simulink model "VCU_CS75_12_30_test"  (R2014a)
settings: Solver=FixedStepDiscrete  StartTime=0.0  StopTime=25  FixedStep=0.0005  RelTol=1e-3
InitFcn:
  | PID_canshu
values from neighbouring files (symbols this model uses):
  D1 = ecucoder_cal(D1)    [PID_canshu.m]
  D2 = ecucoder_cal(D2)    [PID_canshu.m]
  D3 = ecucoder_cal(D3)    [PID_canshu.m]
  ErrorLimit = ecucoder_cal(ErrorLimit)    [PID_canshu.m]
  ErrorSumMax1 = ecucoder_cal(ErrorSumMax1)    [PID_canshu.m]
  ErrorSumMax2 = ecucoder_cal(ErrorSumMax2)    [PID_canshu.m]
  ErrorSumMax3 = ecucoder_cal(ErrorSumMax3)    [PID_canshu.m]
  I1 = ecucoder_cal(I1)    [PID_canshu.m]
  I2 = ecucoder_cal(I2)    [PID_canshu.m]
  I3 = ecucoder_cal(I3)    [PID_canshu.m]
  Limit1 = ecucoder_cal(Limit1)    [PID_canshu.m]
  Limit2 = ecucoder_cal(Limit2)    [PID_canshu.m]
  P1 = ecucoder_cal(P1)    [PID_canshu.m]
  P2 = ecucoder_cal(P2)    [PID_canshu.m]
  P3 = ecucoder_cal(P3)    [PID_canshu.m]
  T_buchang = ecucoder_cal(T_buchang)    [PID_canshu.m]
undefined symbols (not defined in the file or in its folder): ecucoder_acal, I_SW01_L, LaterlAngleCommand, LDW, RemoteAcclPosition
libraries: simulink x940, ec5744lib x41
(part 20 of 31)

== system VCU_CS75_12_30_test/长安CS75底盘程序，20ms一次/Output/Subsystem/TransmitMessages10/LAS_29D/LAS_HostLaneLeftStatus ==
  LAS_HostLaneLeftStatus : Inport
  Constant{1..2,4..8} (7 alike) : Constant  Value=0  OutDataTypeStr=uint8
  LAS_HostLaneLeftStatusRon : Rounding  Operator=round
  LAS_HostLaneLeftStatus_1sat : Saturate  UpperLimit=7  LowerLimit=0
  LAS_HostLaneLeftStatus_Convert : DataTypeConversion  OutDataTypeStr=uint8
  LAS_HostLaneLeftStatus_Convert1 : DataTypeConversion  OutDataTypeStr=uint32
  LAS_HostLaneLeftStatus_D : Product  Inputs=*/
  LAS_HostLaneLeftStatus_F : Constant  OutDataTypeStr=single
  LAS_HostLaneLeftStatus_L : simulink/Logic and Bit Operations/Bitwise Operator  logicop=AND  UseBitMask=on  BitMask=7  BitMaskRealWorld=Stored Integer
  LAS_HostLaneLeftStatus_O : Constant  Value=0  OutDataTypeStr=single
  LAS_HostLaneLeftStatus_S : ArithShift
  LAS_HostLaneLeftStatus_sat : Saturate  UpperLimit=0  LowerLimit=0
  LAS_HostLaneLeftStatus_st : Sum  Inputs=+-
  output1 : Outport
  output2 : Outport  Port=2
  output3 : Outport  Port=3
  output4 : Outport  Port=4
  output5 : Outport  Port=5
  output6 : Outport  Port=6
  output7 : Outport  Port=7
  output8 : Outport  Port=8
  wires:
  LAS_HostLaneLeftStatus/1 -> LAS_HostLaneLeftStatus_sat/1
  LAS_HostLaneLeftStatus_sat/1 -> LAS_HostLaneLeftStatus_st/1
  LAS_HostLaneLeftStatus_O/1 -> LAS_HostLaneLeftStatus_st/2
  LAS_HostLaneLeftStatus_st/1 -> LAS_HostLaneLeftStatus_D/1
  LAS_HostLaneLeftStatus_F/1 -> LAS_HostLaneLeftStatus_D/2
  LAS_HostLaneLeftStatus_D/1 -> LAS_HostLaneLeftStatusRon/1
  LAS_HostLaneLeftStatusRon/1 -> LAS_HostLaneLeftStatus_S/1
  LAS_HostLaneLeftStatus_S/1 -> LAS_HostLaneLeftStatus_1sat/1
  LAS_HostLaneLeftStatus_1sat/1 -> LAS_HostLaneLeftStatus_Convert1/1
  LAS_HostLaneLeftStatus_Convert1/1 -> LAS_HostLaneLeftStatus_L/1
  LAS_HostLaneLeftStatus_L/1 -> LAS_HostLaneLeftStatus_Convert/1
  LAS_HostLaneLeftStatus_Convert/1 -> output3/1
  Constant1/1 -> output1/1
  Constant2/1 -> output2/1
  Constant4/1 -> output4/1
  Constant5/1 -> output5/1
  Constant6/1 -> output6/1
  Constant7/1 -> output7/1
  Constant8/1 -> output8/1

== system VCU_CS75_12_30_test/长安CS75底盘程序，20ms一次/Output/Subsystem/TransmitMessages10/LAS_29D/LAS_HostLaneRightStatus ==
  LAS_HostLaneRightStatus : Inport
  Constant{1..3,5..8} (7 alike) : Constant  Value=0  OutDataTypeStr=uint8
  LAS_HostLaneRightStatusRon : Rounding  Operator=round
  LAS_HostLaneRightStatus_1sat : Saturate  UpperLimit=7  LowerLimit=0
  LAS_HostLaneRightStatus_Convert : DataTypeConversion  OutDataTypeStr=uint8
  LAS_HostLaneRightStatus_Convert1 : DataTypeConversion  OutDataTypeStr=uint32
  LAS_HostLaneRightStatus_D : Product  Inputs=*/
  LAS_HostLaneRightStatus_F : Constant  OutDataTypeStr=single
  LAS_HostLaneRightStatus_L : simulink/Logic and Bit Operations/Bitwise Operator  logicop=AND  UseBitMask=on  BitMask=7  BitMaskRealWorld=Stored Integer
  LAS_HostLaneRightStatus_O : Constant  Value=0  OutDataTypeStr=single
  LAS_HostLaneRightStatus_S : ArithShift
  LAS_HostLaneRightStatus_sat : Saturate  UpperLimit=0  LowerLimit=0
  LAS_HostLaneRightStatus_st : Sum  Inputs=+-
  output1 : Outport
  output2 : Outport  Port=2
  output3 : Outport  Port=3
  output4 : Outport  Port=4
  output5 : Outport  Port=5
  output6 : Outport  Port=6
  output7 : Outport  Port=7
  output8 : Outport  Port=8
  wires:
  LAS_HostLaneRightStatus/1 -> LAS_HostLaneRightStatus_sat/1
  LAS_HostLaneRightStatus_sat/1 -> LAS_HostLaneRightStatus_st/1
  LAS_HostLaneRightStatus_O/1 -> LAS_HostLaneRightStatus_st/2
  LAS_HostLaneRightStatus_st/1 -> LAS_HostLaneRightStatus_D/1
  LAS_HostLaneRightStatus_F/1 -> LAS_HostLaneRightStatus_D/2
  LAS_HostLaneRightStatus_D/1 -> LAS_HostLaneRightStatusRon/1
  LAS_HostLaneRightStatusRon/1 -> LAS_HostLaneRightStatus_S/1
  LAS_HostLaneRightStatus_S/1 -> LAS_HostLaneRightStatus_1sat/1
  LAS_HostLaneRightStatus_1sat/1 -> LAS_HostLaneRightStatus_Convert1/1
  LAS_HostLaneRightStatus_Convert1/1 -> LAS_HostLaneRightStatus_L/1
  LAS_HostLaneRightStatus_L/1 -> LAS_HostLaneRightStatus_Convert/1
  LAS_HostLaneRightStatus_Convert/1 -> output4/1
  Constant1/1 -> output1/1
  Constant2/1 -> output2/1
  Constant3/1 -> output3/1
  Constant5/1 -> output5/1
  Constant6/1 -> output6/1
  Constant7/1 -> output7/1
  Constant8/1 -> output8/1

== system VCU_CS75_12_30_test/长安CS75底盘程序，20ms一次/Output/Subsystem/TransmitMessages10/LAS_29D/LAS_IACCEnableStatus ==
  LAS_IACCEnableStatus : Inport
  Constant{1..6,8} (7 alike) : Constant  Value=0  OutDataTypeStr=uint8
  LAS_IACCEnableStatusRon : Rounding  Operator=round
  LAS_IACCEnableStatus_1sat : Saturate  UpperLimit=48  LowerLimit=0
  LAS_IACCEnableStatus_Convert : DataTypeConversion  OutDataTypeStr=uint8
  LAS_IACCEnableStatus_Convert1 : DataTypeConversion  OutDataTypeStr=uint32
  LAS_IACCEnableStatus_D : Product  Inputs=*/
  LAS_IACCEnableStatus_F : Constant  OutDataTypeStr=single
  LAS_IACCEnableStatus_L : simulink/Logic and Bit Operations/Bitwise Operator  logicop=AND  UseBitMask=on  BitMask=48  BitMaskRealWorld=Stored Integer
  LAS_IACCEnableStatus_O : Constant  Value=0  OutDataTypeStr=single
  LAS_IACCEnableStatus_S : ArithShift  BitShiftNumber=-4
  LAS_IACCEnableStatus_sat : Saturate  UpperLimit=3  LowerLimit=0
  LAS_IACCEnableStatus_st : Sum  Inputs=+-
  output1 : Outport
  output2 : Outport  Port=2
  output3 : Outport  Port=3
  output4 : Outport  Port=4
  output5 : Outport  Port=5
  output6 : Outport  Port=6
  output7 : Outport  Port=7
  output8 : Outport  Port=8
  wires:
  LAS_IACCEnableStatus/1 -> LAS_IACCEnableStatus_sat/1
  LAS_IACCEnableStatus_sat/1 -> LAS_IACCEnableStatus_st/1
  LAS_IACCEnableStatus_O/1 -> LAS_IACCEnableStatus_st/2
  LAS_IACCEnableStatus_st/1 -> LAS_IACCEnableStatus_D/1
  LAS_IACCEnableStatus_F/1 -> LAS_IACCEnableStatus_D/2
  LAS_IACCEnableStatus_D/1 -> LAS_IACCEnableStatusRon/1
  LAS_IACCEnableStatusRon/1 -> LAS_IACCEnableStatus_S/1
  LAS_IACCEnableStatus_S/1 -> LAS_IACCEnableStatus_1sat/1
  LAS_IACCEnableStatus_1sat/1 -> LAS_IACCEnableStatus_Convert1/1
  LAS_IACCEnableStatus_Convert1/1 -> LAS_IACCEnableStatus_L/1
  LAS_IACCEnableStatus_L/1 -> LAS_IACCEnableStatus_Convert/1
  LAS_IACCEnableStatus_Convert/1 -> output7/1
  Constant1/1 -> output1/1
  Constant2/1 -> output2/1
  Constant3/1 -> output3/1
  Constant4/1 -> output4/1
  Constant5/1 -> output5/1
  Constant6/1 -> output6/1
  Constant8/1 -> output8/1

== system VCU_CS75_12_30_test/长安CS75底盘程序，20ms一次/Output/Subsystem/TransmitMessages10/LAS_29D/LAS_LASModeSelectionStatus ==
  LAS_LASModeSelectionStatus : Inport
  Constant{2..8} (7 alike) : Constant  Value=0  OutDataTypeStr=uint8
  LAS_LASModeSelectionStatusRon : Rounding  Operator=round
  LAS_LASModeSelectionStatus_1sat : Saturate  UpperLimit=56  LowerLimit=0
  LAS_LASModeSelectionStatus_Convert : DataTypeConversion  OutDataTypeStr=uint8
  LAS_LASModeSelectionStatus_Convert1 : DataTypeConversion  OutDataTypeStr=uint32
  LAS_LASModeSelectionStatus_D : Product  Inputs=*/
  LAS_LASModeSelectionStatus_F : Constant  OutDataTypeStr=single
  LAS_LASModeSelectionStatus_L : simulink/Logic and Bit Operations/Bitwise Operator  logicop=AND  UseBitMask=on  BitMask=56  BitMaskRealWorld=Stored Integer
  LAS_LASModeSelectionStatus_O : Constant  Value=0  OutDataTypeStr=single
  LAS_LASModeSelectionStatus_S : ArithShift  BitShiftNumber=-3
  LAS_LASModeSelectionStatus_sat : Saturate  UpperLimit=7  LowerLimit=0
  LAS_LASModeSelectionStatus_st : Sum  Inputs=+-
  output1 : Outport
  output2 : Outport  Port=2
  output3 : Outport  Port=3
  output4 : Outport  Port=4
  output5 : Outport  Port=5
  output6 : Outport  Port=6
  output7 : Outport  Port=7
  output8 : Outport  Port=8
  wires:
  LAS_LASModeSelectionStatus/1 -> LAS_LASModeSelectionStatus_sat/1
  LAS_LASModeSelectionStatus_sat/1 -> LAS_LASModeSelectionStatus_st/1
  LAS_LASModeSelectionStatus_O/1 -> LAS_LASModeSelectionStatus_st/2
  LAS_LASModeSelectionStatus_st/1 -> LAS_LASModeSelectionStatus_D/1
  LAS_LASModeSelectionStatus_F/1 -> LAS_LASModeSelectionStatus_D/2
  LAS_LASModeSelectionStatus_D/1 -> LAS_LASModeSelectionStatusRon/1
  LAS_LASModeSelectionStatusRon/1 -> LAS_LASModeSelectionStatus_S/1
  LAS_LASModeSelectionStatus_S/1 -> LAS_LASModeSelectionStatus_1sat/1
  LAS_LASModeSelectionStatus_1sat/1 -> LAS_LASModeSelectionStatus_Convert1/1
  LAS_LASModeSelectionStatus_Convert1/1 -> LAS_LASModeSelectionStatus_L/1
  LAS_LASModeSelectionStatus_L/1 -> LAS_LASModeSelectionStatus_Convert/1
  LAS_LASModeSelectionStatus_Convert/1 -> output1/1
  Constant2/1 -> output2/1
  Constant3/1 -> output3/1
  Constant4/1 -> output4/1
  Constant5/1 -> output5/1
  Constant6/1 -> output6/1
  Constant7/1 -> output7/1
  Constant8/1 -> output8/1

== system VCU_CS75_12_30_test/长安CS75底盘程序，20ms一次/Output/Subsystem/TransmitMessages10/LAS_29D/LAS_LASWarningModeSelectionSts ==
  LAS_LASWarningModeSelectionSts : Inport
  Constant{3..8} (6 alike) : Constant  Value=0  OutDataTypeStr=uint8
  LAS_LASWarningModeSelectionStsBitCov : DataTypeConversion  OutDataTypeStr=uint8
  LAS_LASWarningModeSelectionStsCOV : DataTypeConversion  OutDataTypeStr=uint8
  LAS_LASWarningModeSelectionStsRon : Rounding  Operator=round
  LAS_LASWarningModeSelectionSts_1sat : Saturate  UpperLimit=448  LowerLimit=0
  LAS_LASWarningModeSelectionSts_And : simulink/Logic and Bit Operations/Bitwise Operator  logicop=AND  UseBitMask=off  NumInputPorts=2  BitMask=bin2dec('11011001')  BitMaskRealWorld=Stored Integer
  LAS_LASWarningModeSelectionSts_And_C : Constant  Value=255  OutDataTypeStr=uint32
  LAS_LASWarningModeSelectionSts_Convert : DataTypeConversion  OutDataTypeStr=uint32
  LAS_LASWarningModeSelectionSts_D : Product  Inputs=*/
  LAS_LASWarningModeSelectionSts_D1 : Product  Inputs=*/
  LAS_LASWarningModeSelectionSts_F : Constant  OutDataTypeStr=single
  LAS_LASWarningModeSelectionSts_L : simulink/Logic and Bit Operations/Bitwise Operator  logicop=AND  UseBitMask=on  BitMask=448  BitMaskRealWorld=Stored Integer
  LAS_LASWarningModeSelectionSts_O : Constant  Value=0  OutDataTypeStr=single
  LAS_LASWarningModeSelectionSts_S : ArithShift  BitShiftNumber=-6
  LAS_LASWarningModeSelectionSts_sat : Saturate  UpperLimit=7  LowerLimit=0
  LAS_LASWarningModeSelectionSts_st : Sum  Inputs=+-
  LAS_LASWarningModeSelectionStsoutput1_C : Constant  Value=256
  output1 : Outport
  output2 : Outport  Port=2
  output3 : Outport  Port=3
  output4 : Outport  Port=4
  output5 : Outport  Port=5
  output6 : Outport  Port=6
  output7 : Outport  Port=7
  output8 : Outport  Port=8
  wires:
  LAS_LASWarningModeSelectionSts/1 -> LAS_LASWarningModeSelectionSts_sat/1
  LAS_LASWarningModeSelectionSts_sat/1 -> LAS_LASWarningModeSelectionSts_st/1
  LAS_LASWarningModeSelectionSts_O/1 -> LAS_LASWarningModeSelectionSts_st/2
  LAS_LASWarningModeSelectionSts_st/1 -> LAS_LASWarningModeSelectionSts_D/1
  LAS_LASWarningModeSelectionSts_F/1 -> LAS_LASWarningModeSelectionSts_D/2
  LAS_LASWarningModeSelectionSts_D/1 -> LAS_LASWarningModeSelectionStsRon/1
  LAS_LASWarningModeSelectionStsRon/1 -> LAS_LASWarningModeSelectionSts_S/1
  LAS_LASWarningModeSelectionSts_S/1 -> LAS_LASWarningModeSelectionSts_1sat/1
  LAS_LASWarningModeSelectionSts_1sat/1 -> LAS_LASWarningModeSelectionSts_Convert/1
  LAS_LASWarningModeSelectionSts_Convert/1 -> LAS_LASWarningModeSelectionSts_L/1
  LAS_LASWarningModeSelectionSts_L/1 -> LAS_LASWarningModeSelectionSts_D1/1, LAS_LASWarningModeSelectionSts_And/1
  LAS_LASWarningModeSelectionStsoutput1_C/1 -> LAS_LASWarningModeSelectionSts_D1/2
  LAS_LASWarningModeSelectionSts_D1/1 -> LAS_LASWarningModeSelectionStsCOV/1
  LAS_LASWarningModeSelectionStsCOV/1 -> output1/1
  LAS_LASWarningModeSelectionSts_And_C/1 -> LAS_LASWarningModeSelectionSts_And/2
  LAS_LASWarningModeSelectionSts_And/1 -> LAS_LASWarningModeSelectionStsBitCov/1
  LAS_LASWarningModeSelectionStsBitCov/1 -> output2/1
  Constant3/1 -> output3/1
  Constant4/1 -> output4/1
  Constant5/1 -> output5/1
  Constant6/1 -> output6/1
  Constant7/1 -> output7/1
  Constant8/1 -> output8/1

== system VCU_CS75_12_30_test/长安CS75底盘程序，20ms一次/Output/Subsystem/TransmitMessages10/LAS_29D/LAS_LDWShakeLevStatus ==
  LAS_LDWShakeLevStatus : Inport
  Constant{1,3..8} (7 alike) : Constant  Value=0  OutDataTypeStr=uint8
  LAS_LDWShakeLevStatusRon : Rounding  Operator=round
  LAS_LDWShakeLevStatus_1sat : Saturate  UpperLimit=48  LowerLimit=0
  LAS_LDWShakeLevStatus_Convert : DataTypeConversion  OutDataTypeStr=uint8
  LAS_LDWShakeLevStatus_Convert1 : DataTypeConversion  OutDataTypeStr=uint32
  LAS_LDWShakeLevStatus_D : Product  Inputs=*/
  LAS_LDWShakeLevStatus_F : Constant  OutDataTypeStr=single
  LAS_LDWShakeLevStatus_L : simulink/Logic and Bit Operations/Bitwise Operator  logicop=AND  UseBitMask=on  BitMask=48  BitMaskRealWorld=Stored Integer
  LAS_LDWShakeLevStatus_O : Constant  Value=0  OutDataTypeStr=single
  LAS_LDWShakeLevStatus_S : ArithShift  BitShiftNumber=-4
  LAS_LDWShakeLevStatus_sat : Saturate  UpperLimit=3  LowerLimit=0
  LAS_LDWShakeLevStatus_st : Sum  Inputs=+-
  output1 : Outport
  output2 : Outport  Port=2
  output3 : Outport  Port=3
  output4 : Outport  Port=4
  output5 : Outport  Port=5
  output6 : Outport  Port=6
  output7 : Outport  Port=7
  output8 : Outport  Port=8
  wires:
  LAS_LDWShakeLevStatus/1 -> LAS_LDWShakeLevStatus_sat/1
  LAS_LDWShakeLevStatus_sat/1 -> LAS_LDWShakeLevStatus_st/1
  LAS_LDWShakeLevStatus_O/1 -> LAS_LDWShakeLevStatus_st/2
  LAS_LDWShakeLevStatus_st/1 -> LAS_LDWShakeLevStatus_D/1
  LAS_LDWShakeLevStatus_F/1 -> LAS_LDWShakeLevStatus_D/2
  LAS_LDWShakeLevStatus_D/1 -> LAS_LDWShakeLevStatusRon/1
  LAS_LDWShakeLevStatusRon/1 -> LAS_LDWShakeLevStatus_S/1
  LAS_LDWShakeLevStatus_S/1 -> LAS_LDWShakeLevStatus_1sat/1
  LAS_LDWShakeLevStatus_1sat/1 -> LAS_LDWShakeLevStatus_Convert1/1
  LAS_LDWShakeLevStatus_Convert1/1 -> LAS_LDWShakeLevStatus_L/1
  LAS_LDWShakeLevStatus_L/1 -> LAS_LDWShakeLevStatus_Convert/1
  LAS_LDWShakeLevStatus_Convert/1 -> output2/1
  Constant1/1 -> output1/1
  Constant3/1 -> output3/1
  Constant4/1 -> output4/1
  Constant5/1 -> output5/1
  Constant6/1 -> output6/1
  Constant7/1 -> output7/1
  Constant8/1 -> output8/1

== system VCU_CS75_12_30_test/长安CS75底盘程序，20ms一次/Output/Subsystem/TransmitMessages10/LAS_29D/LAS_LLaneMarkerType ==
  LAS_LLaneMarkerType : Inport
  Constant{1..4,6..8} (7 alike) : Constant  Value=0  OutDataTypeStr=uint8
  LAS_LLaneMarkerTypeRon : Rounding  Operator=round
  LAS_LLaneMarkerType_1sat : Saturate  UpperLimit=7  LowerLimit=0
  LAS_LLaneMarkerType_Convert : DataTypeConversion  OutDataTypeStr=uint8
  LAS_LLaneMarkerType_Convert1 : DataTypeConversion  OutDataTypeStr=uint32
  LAS_LLaneMarkerType_D : Product  Inputs=*/
  LAS_LLaneMarkerType_F : Constant  OutDataTypeStr=single
  LAS_LLaneMarkerType_L : simulink/Logic and Bit Operations/Bitwise Operator  logicop=AND  UseBitMask=on  BitMask=7  BitMaskRealWorld=Stored Integer
  LAS_LLaneMarkerType_O : Constant  Value=0  OutDataTypeStr=single
  LAS_LLaneMarkerType_S : ArithShift
  LAS_LLaneMarkerType_sat : Saturate  UpperLimit=7  LowerLimit=0
  LAS_LLaneMarkerType_st : Sum  Inputs=+-
  output1 : Outport
  output2 : Outport  Port=2
  output3 : Outport  Port=3
  output4 : Outport  Port=4
  output5 : Outport  Port=5
  output6 : Outport  Port=6
  output7 : Outport  Port=7
  output8 : Outport  Port=8
  wires:
  LAS_LLaneMarkerType/1 -> LAS_LLaneMarkerType_sat/1
  LAS_LLaneMarkerType_sat/1 -> LAS_LLaneMarkerType_st/1
  LAS_LLaneMarkerType_O/1 -> LAS_LLaneMarkerType_st/2
  LAS_LLaneMarkerType_st/1 -> LAS_LLaneMarkerType_D/1
  LAS_LLaneMarkerType_F/1 -> LAS_LLaneMarkerType_D/2
  LAS_LLaneMarkerType_D/1 -> LAS_LLaneMarkerTypeRon/1
  LAS_LLaneMarkerTypeRon/1 -> LAS_LLaneMarkerType_S/1
  LAS_LLaneMarkerType_S/1 -> LAS_LLaneMarkerType_1sat/1
  LAS_LLaneMarkerType_1sat/1 -> LAS_LLaneMarkerType_Convert1/1
  LAS_LLaneMarkerType_Convert1/1 -> LAS_LLaneMarkerType_L/1
  LAS_LLaneMarkerType_L/1 -> LAS_LLaneMarkerType_Convert/1
  LAS_LLaneMarkerType_Convert/1 -> output5/1
  Constant1/1 -> output1/1
  Constant2/1 -> output2/1
  Constant3/1 -> output3/1
  Constant4/1 -> output4/1
  Constant6/1 -> output6/1
  Constant7/1 -> output7/1
  Constant8/1 -> output8/1

== system VCU_CS75_12_30_test/长安CS75底盘程序，20ms一次/Output/Subsystem/TransmitMessages10/LAS_29D/LAS_LdwSensitivityStatus ==
  LAS_LdwSensitivityStatus : Inport
  Constant{2..8} (7 alike) : Constant  Value=0  OutDataTypeStr=uint8
  LAS_LdwSensitivityStatusRon : Rounding  Operator=round
  LAS_LdwSensitivityStatus_1sat : Saturate  UpperLimit=192  LowerLimit=0
  LAS_LdwSensitivityStatus_Convert : DataTypeConversion  OutDataTypeStr=uint8
  LAS_LdwSensitivityStatus_Convert1 : DataTypeConversion  OutDataTypeStr=uint32
  LAS_LdwSensitivityStatus_D : Product  Inputs=*/
  LAS_LdwSensitivityStatus_F : Constant  OutDataTypeStr=single
  LAS_LdwSensitivityStatus_L : simulink/Logic and Bit Operations/Bitwise Operator  logicop=AND  UseBitMask=on  BitMask=192  BitMaskRealWorld=Stored Integer
  LAS_LdwSensitivityStatus_O : Constant  Value=0  OutDataTypeStr=single
  LAS_LdwSensitivityStatus_S : ArithShift  BitShiftNumber=-6
  LAS_LdwSensitivityStatus_sat : Saturate  UpperLimit=3  LowerLimit=0
  LAS_LdwSensitivityStatus_st : Sum  Inputs=+-
  output1 : Outport
  output2 : Outport  Port=2
  output3 : Outport  Port=3
  output4 : Outport  Port=4
  output5 : Outport  Port=5
  output6 : Outport  Port=6
  output7 : Outport  Port=7
  output8 : Outport  Port=8
  wires:
  LAS_LdwSensitivityStatus/1 -> LAS_LdwSensitivityStatus_sat/1
  LAS_LdwSensitivityStatus_sat/1 -> LAS_LdwSensitivityStatus_st/1
  LAS_LdwSensitivityStatus_O/1 -> LAS_LdwSensitivityStatus_st/2
  LAS_LdwSensitivityStatus_st/1 -> LAS_LdwSensitivityStatus_D/1
  LAS_LdwSensitivityStatus_F/1 -> LAS_LdwSensitivityStatus_D/2
  LAS_LdwSensitivityStatus_D/1 -> LAS_LdwSensitivityStatusRon/1
  LAS_LdwSensitivityStatusRon/1 -> LAS_LdwSensitivityStatus_S/1
  LAS_LdwSensitivityStatus_S/1 -> LAS_LdwSensitivityStatus_1sat/1
  LAS_LdwSensitivityStatus_1sat/1 -> LAS_LdwSensitivityStatus_Convert1/1
  LAS_LdwSensitivityStatus_Convert1/1 -> LAS_LdwSensitivityStatus_L/1
  LAS_LdwSensitivityStatus_L/1 -> LAS_LdwSensitivityStatus_Convert/1
  LAS_LdwSensitivityStatus_Convert/1 -> output1/1
  Constant2/1 -> output2/1
  Constant3/1 -> output3/1
  Constant4/1 -> output4/1
  Constant5/1 -> output5/1
  Constant6/1 -> output6/1
  Constant7/1 -> output7/1
  Constant8/1 -> output8/1

== system VCU_CS75_12_30_test/长安CS75底盘程序，20ms一次/Output/Subsystem/TransmitMessages10/LAS_29D/LAS_OverspeedSoundWarning ==
  LAS_OverspeedSoundWarning : Inport
  Constant{1..3,5..8} (7 alike) : Constant  Value=0  OutDataTypeStr=uint8
  LAS_OverspeedSoundWarningRon : Rounding  Operator=round
  LAS_OverspeedSoundWarning_1sat : Saturate  UpperLimit=192  LowerLimit=0
  LAS_OverspeedSoundWarning_Convert : DataTypeConversion  OutDataTypeStr=uint8
  LAS_OverspeedSoundWarning_Convert1 : DataTypeConversion  OutDataTypeStr=uint32
  LAS_OverspeedSoundWarning_D : Product  Inputs=*/
  LAS_OverspeedSoundWarning_F : Constant  OutDataTypeStr=single
  LAS_OverspeedSoundWarning_L : simulink/Logic and Bit Operations/Bitwise Operator  logicop=AND  UseBitMask=on  BitMask=192  BitMaskRealWorld=Stored Integer
  LAS_OverspeedSoundWarning_O : Constant  Value=0  OutDataTypeStr=single
  LAS_OverspeedSoundWarning_S : ArithShift  BitShiftNumber=-6
  LAS_OverspeedSoundWarning_sat : Saturate  UpperLimit=3  LowerLimit=0
  LAS_OverspeedSoundWarning_st : Sum  Inputs=+-
  output1 : Outport
  output2 : Outport  Port=2
  output3 : Outport  Port=3
  output4 : Outport  Port=4
  output5 : Outport  Port=5
  output6 : Outport  Port=6
  output7 : Outport  Port=7
  output8 : Outport  Port=8
  wires:
  LAS_OverspeedSoundWarning/1 -> LAS_OverspeedSoundWarning_sat/1
  LAS_OverspeedSoundWarning_sat/1 -> LAS_OverspeedSoundWarning_st/1
  LAS_OverspeedSoundWarning_O/1 -> LAS_OverspeedSoundWarning_st/2
  LAS_OverspeedSoundWarning_st/1 -> LAS_OverspeedSoundWarning_D/1
  LAS_OverspeedSoundWarning_F/1 -> LAS_OverspeedSoundWarning_D/2
  LAS_OverspeedSoundWarning_D/1 -> LAS_OverspeedSoundWarningRon/1
  LAS_OverspeedSoundWarningRon/1 -> LAS_OverspeedSoundWarning_S/1
  LAS_OverspeedSoundWarning_S/1 -> LAS_OverspeedSoundWarning_1sat/1
  LAS_OverspeedSoundWarning_1sat/1 -> LAS_OverspeedSoundWarning_Convert1/1
  LAS_OverspeedSoundWarning_Convert1/1 -> LAS_OverspeedSoundWarning_L/1
  LAS_OverspeedSoundWarning_L/1 -> LAS_OverspeedSoundWarning_Convert/1
  LAS_OverspeedSoundWarning_Convert/1 -> output4/1
  Constant1/1 -> output1/1
  Constant2/1 -> output2/1
  Constant3/1 -> output3/1
  Constant5/1 -> output5/1
  Constant6/1 -> output6/1
  Constant7/1 -> output7/1
  Constant8/1 -> output8/1

== system VCU_CS75_12_30_test/长安CS75底盘程序，20ms一次/Output/Subsystem/TransmitMessages10/LAS_29D/LAS_OverspeedSoundWarningEnSt ==
  LAS_OverspeedSoundWarningEnSt : Inport
  Constant{1,3..8} (7 alike) : Constant  Value=0  OutDataTypeStr=uint8
  LAS_OverspeedSoundWarningEnStRon : Rounding  Operator=round
  LAS_OverspeedSoundWarningEnSt_1sat : Saturate  UpperLimit=3  LowerLimit=0
  LAS_OverspeedSoundWarningEnSt_Convert : DataTypeConversion  OutDataTypeStr=uint8
  LAS_OverspeedSoundWarningEnSt_Convert1 : DataTypeConversion  OutDataTypeStr=uint32
  LAS_OverspeedSoundWarningEnSt_D : Product  Inputs=*/
  LAS_OverspeedSoundWarningEnSt_F : Constant  OutDataTypeStr=single
  LAS_OverspeedSoundWarningEnSt_L : simulink/Logic and Bit Operations/Bitwise Operator  logicop=AND  UseBitMask=on  BitMask=3  BitMaskRealWorld=Stored Integer
  LAS_OverspeedSoundWarningEnSt_O : Constant  Value=0  OutDataTypeStr=single
  LAS_OverspeedSoundWarningEnSt_S : ArithShift
  LAS_OverspeedSoundWarningEnSt_sat : Saturate  UpperLimit=3  LowerLimit=0
  LAS_OverspeedSoundWarningEnSt_st : Sum  Inputs=+-
  output1 : Outport
  output2 : Outport  Port=2
  output3 : Outport  Port=3
  output4 : Outport  Port=4
  output5 : Outport  Port=5
  output6 : Outport  Port=6
  output7 : Outport  Port=7
  output8 : Outport  Port=8
  wires:
  LAS_OverspeedSoundWarningEnSt/1 -> LAS_OverspeedSoundWarningEnSt_sat/1
  LAS_OverspeedSoundWarningEnSt_sat/1 -> LAS_OverspeedSoundWarningEnSt_st/1
  LAS_OverspeedSoundWarningEnSt_O/1 -> LAS_OverspeedSoundWarningEnSt_st/2
  LAS_OverspeedSoundWarningEnSt_st/1 -> LAS_OverspeedSoundWarningEnSt_D/1
  LAS_OverspeedSoundWarningEnSt_F/1 -> LAS_OverspeedSoundWarningEnSt_D/2
  LAS_OverspeedSoundWarningEnSt_D/1 -> LAS_OverspeedSoundWarningEnStRon/1
  LAS_OverspeedSoundWarningEnStRon/1 -> LAS_OverspeedSoundWarningEnSt_S/1
  LAS_OverspeedSoundWarningEnSt_S/1 -> LAS_OverspeedSoundWarningEnSt_1sat/1
  LAS_OverspeedSoundWarningEnSt_1sat/1 -> LAS_OverspeedSoundWarningEnSt_Convert1/1
  LAS_OverspeedSoundWarningEnSt_Convert1/1 -> LAS_OverspeedSoundWarningEnSt_L/1
  LAS_OverspeedSoundWarningEnSt_L/1 -> LAS_OverspeedSoundWarningEnSt_Convert/1
  LAS_OverspeedSoundWarningEnSt_Convert/1 -> output2/1
  Constant1/1 -> output1/1
  Constant3/1 -> output3/1
  Constant4/1 -> output4/1
  Constant5/1 -> output5/1
  Constant6/1 -> output6/1
  Constant7/1 -> output7/1
  Constant8/1 -> output8/1

== system VCU_CS75_12_30_test/长安CS75底盘程序，20ms一次/Output/Subsystem/TransmitMessages10/LAS_29D/LAS_OverspeedVisualWarning ==
  LAS_OverspeedVisualWarning : Inport
  Constant{1..4,6..8} (7 alike) : Constant  Value=0  OutDataTypeStr=uint8
  LAS_OverspeedVisualWarningRon : Rounding  Operator=round
  LAS_OverspeedVisualWarning_1sat : Saturate  UpperLimit=192  LowerLimit=0
  LAS_OverspeedVisualWarning_Convert : DataTypeConversion  OutDataTypeStr=uint8
  LAS_OverspeedVisualWarning_Convert1 : DataTypeConversion  OutDataTypeStr=uint32
  LAS_OverspeedVisualWarning_D : Product  Inputs=*/
  LAS_OverspeedVisualWarning_F : Constant  OutDataTypeStr=single
  LAS_OverspeedVisualWarning_L : simulink/Logic and Bit Operations/Bitwise Operator  logicop=AND  UseBitMask=on  BitMask=192  BitMaskRealWorld=Stored Integer
  LAS_OverspeedVisualWarning_O : Constant  Value=0  OutDataTypeStr=single
  LAS_OverspeedVisualWarning_S : ArithShift  BitShiftNumber=-6
  LAS_OverspeedVisualWarning_sat : Saturate  UpperLimit=3  LowerLimit=0
  LAS_OverspeedVisualWarning_st : Sum  Inputs=+-
  output1 : Outport
  output2 : Outport  Port=2
  output3 : Outport  Port=3
  output4 : Outport  Port=4
  output5 : Outport  Port=5
  output6 : Outport  Port=6
  output7 : Outport  Port=7
  output8 : Outport  Port=8
  wires:
  LAS_OverspeedVisualWarning/1 -> LAS_OverspeedVisualWarning_sat/1
  LAS_OverspeedVisualWarning_sat/1 -> LAS_OverspeedVisualWarning_st/1
  LAS_OverspeedVisualWarning_O/1 -> LAS_OverspeedVisualWarning_st/2
  LAS_OverspeedVisualWarning_st/1 -> LAS_OverspeedVisualWarning_D/1
  LAS_OverspeedVisualWarning_F/1 -> LAS_OverspeedVisualWarning_D/2
  LAS_OverspeedVisualWarning_D/1 -> LAS_OverspeedVisualWarningRon/1
  LAS_OverspeedVisualWarningRon/1 -> LAS_OverspeedVisualWarning_S/1
  LAS_OverspeedVisualWarning_S/1 -> LAS_OverspeedVisualWarning_1sat/1
  LAS_OverspeedVisualWarning_1sat/1 -> LAS_OverspeedVisualWarning_Convert1/1
  LAS_OverspeedVisualWarning_Convert1/1 -> LAS_OverspeedVisualWarning_L/1
  LAS_OverspeedVisualWarning_L/1 -> LAS_OverspeedVisualWarning_Convert/1
  LAS_OverspeedVisualWarning_Convert/1 -> output5/1
  Constant1/1 -> output1/1
  Constant2/1 -> output2/1
  Constant3/1 -> output3/1
  Constant4/1 -> output4/1
  Constant6/1 -> output6/1
  Constant7/1 -> output7/1
  Constant8/1 -> output8/1

== system VCU_CS75_12_30_test/长安CS75底盘程序，20ms一次/Output/Subsystem/TransmitMessages10/LAS_29D/LAS_OverspeedWarningEnableStatus ==
  LAS_OverspeedWarningEnableStatus : Inport
  Constant{1..3,5..8} (7 alike) : Constant  Value=0  OutDataTypeStr=uint8
  LAS_OverspeedWarningEnableStatusRon : Rounding  Operator=round
  LAS_OverspeedWarningEnableStatus_1sat : Saturate  UpperLimit=48  LowerLimit=0
  LAS_OverspeedWarningEnableStatus_Convert : DataTypeConversion  OutDataTypeStr=uint8
  LAS_OverspeedWarningEnableStatus_Convert1 : DataTypeConversion  OutDataTypeStr=uint32
  LAS_OverspeedWarningEnableStatus_D : Product  Inputs=*/
  LAS_OverspeedWarningEnableStatus_F : Constant  OutDataTypeStr=single
  LAS_OverspeedWarningEnableStatus_L : simulink/Logic and Bit Operations/Bitwise Operator  logicop=AND  UseBitMask=on  BitMask=48  BitMaskRealWorld=Stored Integer
  LAS_OverspeedWarningEnableStatus_O : Constant  Value=0  OutDataTypeStr=single
  LAS_OverspeedWarningEnableStatus_S : ArithShift  BitShiftNumber=-4
  LAS_OverspeedWarningEnableStatus_sat : Saturate  UpperLimit=3  LowerLimit=0
  LAS_OverspeedWarningEnableStatus_st : Sum  Inputs=+-
  output1 : Outport
  output2 : Outport  Port=2
  output3 : Outport  Port=3
  output4 : Outport  Port=4
  output5 : Outport  Port=5
  output6 : Outport  Port=6
  output7 : Outport  Port=7
  output8 : Outport  Port=8
  wires:
  LAS_OverspeedWarningEnableStatus/1 -> LAS_OverspeedWarningEnableStatus_sat/1
  LAS_OverspeedWarningEnableStatus_sat/1 -> LAS_OverspeedWarningEnableStatus_st/1
  LAS_OverspeedWarningEnableStatus_O/1 -> LAS_OverspeedWarningEnableStatus_st/2
  LAS_OverspeedWarningEnableStatus_st/1 -> LAS_OverspeedWarningEnableStatus_D/1
  LAS_OverspeedWarningEnableStatus_F/1 -> LAS_OverspeedWarningEnableStatus_D/2
  LAS_OverspeedWarningEnableStatus_D/1 -> LAS_OverspeedWarningEnableStatusRon/1
  LAS_OverspeedWarningEnableStatusRon/1 -> LAS_OverspeedWarningEnableStatus_S/1
  LAS_OverspeedWarningEnableStatus_S/1 -> LAS_OverspeedWarningEnableStatus_1sat/1
  LAS_OverspeedWarningEnableStatus_1sat/1 -> LAS_OverspeedWarningEnableStatus_Convert1/1
  LAS_OverspeedWarningEnableStatus_Convert1/1 -> LAS_OverspeedWarningEnableStatus_L/1
  LAS_OverspeedWarningEnableStatus_L/1 -> LAS_OverspeedWarningEnableStatus_Convert/1
  LAS_OverspeedWarningEnableStatus_Convert/1 -> output4/1
  Constant1/1 -> output1/1
  Constant2/1 -> output2/1
  Constant3/1 -> output3/1
  Constant5/1 -> output5/1
  Constant6/1 -> output6/1
  Constant7/1 -> output7/1
  Constant8/1 -> output8/1

== system VCU_CS75_12_30_test/长安CS75底盘程序，20ms一次/Output/Subsystem/TransmitMessages10/LAS_29D/LAS_OverspeedWarningOffset ==
  LAS_OverspeedWarningOffset : Inport
  Constant{1..5,7..8} (7 alike) : Constant  Value=0  OutDataTypeStr=uint8
  LAS_OverspeedWarningOffsetRon : Rounding  Operator=round
  LAS_OverspeedWarningOffset_1sat : Saturate  UpperLimit=248  LowerLimit=0
  LAS_OverspeedWarningOffset_Convert : DataTypeConversion  OutDataTypeStr=uint8
  LAS_OverspeedWarningOffset_Convert1 : DataTypeConversion  OutDataTypeStr=uint32
  LAS_OverspeedWarningOffset_D : Product  Inputs=*/
  LAS_OverspeedWarningOffset_F : Constant  OutDataTypeStr=single
  LAS_OverspeedWarningOffset_L : simulink/Logic and Bit Operations/Bitwise Operator  logicop=AND  UseBitMask=on  BitMask=248  BitMaskRealWorld=Stored Integer
  LAS_OverspeedWarningOffset_O : Constant  Value=-10  OutDataTypeStr=single
  LAS_OverspeedWarningOffset_S : ArithShift  BitShiftNumber=-3
  LAS_OverspeedWarningOffset_sat : Saturate  UpperLimit=10  LowerLimit=-10
  LAS_OverspeedWarningOffset_st : Sum  Inputs=+-
  output1 : Outport
  output2 : Outport  Port=2
  output3 : Outport  Port=3
  output4 : Outport  Port=4
  output5 : Outport  Port=5
  output6 : Outport  Port=6
  output7 : Outport  Port=7
  output8 : Outport  Port=8
  wires:
  LAS_OverspeedWarningOffset/1 -> LAS_OverspeedWarningOffset_sat/1
  LAS_OverspeedWarningOffset_sat/1 -> LAS_OverspeedWarningOffset_st/1
  LAS_OverspeedWarningOffset_O/1 -> LAS_OverspeedWarningOffset_st/2
  LAS_OverspeedWarningOffset_st/1 -> LAS_OverspeedWarningOffset_D/1
  LAS_OverspeedWarningOffset_F/1 -> LAS_OverspeedWarningOffset_D/2
  LAS_OverspeedWarningOffset_D/1 -> LAS_OverspeedWarningOffsetRon/1
  LAS_OverspeedWarningOffsetRon/1 -> LAS_OverspeedWarningOffset_S/1
  LAS_OverspeedWarningOffset_S/1 -> LAS_OverspeedWarningOffset_1sat/1
  LAS_OverspeedWarningOffset_1sat/1 -> LAS_OverspeedWarningOffset_Convert1/1
  LAS_OverspeedWarningOffset_Convert1/1 -> LAS_OverspeedWarningOffset_L/1
  LAS_OverspeedWarningOffset_L/1 -> LAS_OverspeedWarningOffset_Convert/1
  LAS_OverspeedWarningOffset_Convert/1 -> output6/1
  Constant1/1 -> output1/1
  Constant2/1 -> output2/1
  Constant3/1 -> output3/1
  Constant4/1 -> output4/1
  Constant5/1 -> output5/1
  Constant7/1 -> output7/1
  Constant8/1 -> output8/1

== system VCU_CS75_12_30_test/长安CS75底盘程序，20ms一次/Output/Subsystem/TransmitMessages10/LAS_29D/LAS_RLaneMarkerType ==
  LAS_RLaneMarkerType : Inport
  Constant{1..5,7..8} (7 alike) : Constant  Value=0  OutDataTypeStr=uint8
  LAS_RLaneMarkerTypeRon : Rounding  Operator=round
  LAS_RLaneMarkerType_1sat : Saturate  UpperLimit=7  LowerLimit=0
  LAS_RLaneMarkerType_Convert : DataTypeConversion  OutDataTypeStr=uint8
  LAS_RLaneMarkerType_Convert1 : DataTypeConversion  OutDataTypeStr=uint32
  LAS_RLaneMarkerType_D : Product  Inputs=*/
  LAS_RLaneMarkerType_F : Constant  OutDataTypeStr=single
  LAS_RLaneMarkerType_L : simulink/Logic and Bit Operations/Bitwise Operator  logicop=AND  UseBitMask=on  BitMask=7  BitMaskRealWorld=Stored Integer
  LAS_RLaneMarkerType_O : Constant  Value=0  OutDataTypeStr=single
  LAS_RLaneMarkerType_S : ArithShift
  LAS_RLaneMarkerType_sat : Saturate  UpperLimit=7  LowerLimit=0
  LAS_RLaneMarkerType_st : Sum  Inputs=+-
  output1 : Outport
  output2 : Outport  Port=2
  output3 : Outport  Port=3
  output4 : Outport  Port=4
  output5 : Outport  Port=5
  output6 : Outport  Port=6
  output7 : Outport  Port=7
  output8 : Outport  Port=8
  wires:
  LAS_RLaneMarkerType/1 -> LAS_RLaneMarkerType_sat/1
  LAS_RLaneMarkerType_sat/1 -> LAS_RLaneMarkerType_st/1
  LAS_RLaneMarkerType_O/1 -> LAS_RLaneMarkerType_st/2
  LAS_RLaneMarkerType_st/1 -> LAS_RLaneMarkerType_D/1
  LAS_RLaneMarkerType_F/1 -> LAS_RLaneMarkerType_D/2
  LAS_RLaneMarkerType_D/1 -> LAS_RLaneMarkerTypeRon/1
  LAS_RLaneMarkerTypeRon/1 -> LAS_RLaneMarkerType_S/1
  LAS_RLaneMarkerType_S/1 -> LAS_RLaneMarkerType_1sat/1
  LAS_RLaneMarkerType_1sat/1 -> LAS_RLaneMarkerType_Convert1/1
  LAS_RLaneMarkerType_Convert1/1 -> LAS_RLaneMarkerType_L/1
  LAS_RLaneMarkerType_L/1 -> LAS_RLaneMarkerType_Convert/1
  LAS_RLaneMarkerType_Convert/1 -> output6/1
  Constant1/1 -> output1/1
  Constant2/1 -> output2/1
  Constant3/1 -> output3/1
  Constant4/1 -> output4/1
  Constant5/1 -> output5/1
  Constant7/1 -> output7/1
  Constant8/1 -> output8/1

== system VCU_CS75_12_30_test/长安CS75底盘程序，20ms一次/Output/Subsystem/TransmitMessages10/LAS_29D/LAS_SLASwitchStatus ==
  LAS_SLASwitchStatus : Inport
  Constant{2..8} (7 alike) : Constant  Value=0  OutDataTypeStr=uint8
  LAS_SLASwitchStatusRon : Rounding  Operator=round
  LAS_SLASwitchStatus_1sat : Saturate  UpperLimit=2  LowerLimit=0
  LAS_SLASwitchStatus_Convert : DataTypeConversion  OutDataTypeStr=uint8
  LAS_SLASwitchStatus_Convert1 : DataTypeConversion  OutDataTypeStr=uint32
  LAS_SLASwitchStatus_D : Product  Inputs=*/
  LAS_SLASwitchStatus_F : Constant  OutDataTypeStr=single
  LAS_SLASwitchStatus_L : simulink/Logic and Bit Operations/Bitwise Operator  logicop=AND  UseBitMask=on  BitMask=2  BitMaskRealWorld=Stored Integer
  LAS_SLASwitchStatus_O : Constant  Value=0  OutDataTypeStr=single
  LAS_SLASwitchStatus_S : ArithShift  BitShiftNumber=-1
  LAS_SLASwitchStatus_sat : Saturate  UpperLimit=1  LowerLimit=0
  LAS_SLASwitchStatus_st : Sum  Inputs=+-
  output1 : Outport
  output2 : Outport  Port=2
  output3 : Outport  Port=3
  output4 : Outport  Port=4
  output5 : Outport  Port=5
  output6 : Outport  Port=6
  output7 : Outport  Port=7
  output8 : Outport  Port=8
  wires:
  LAS_SLASwitchStatus/1 -> LAS_SLASwitchStatus_sat/1
  LAS_SLASwitchStatus_sat/1 -> LAS_SLASwitchStatus_st/1
  LAS_SLASwitchStatus_O/1 -> LAS_SLASwitchStatus_st/2
  LAS_SLASwitchStatus_st/1 -> LAS_SLASwitchStatus_D/1
  LAS_SLASwitchStatus_F/1 -> LAS_SLASwitchStatus_D/2
  LAS_SLASwitchStatus_D/1 -> LAS_SLASwitchStatusRon/1
  LAS_SLASwitchStatusRon/1 -> LAS_SLASwitchStatus_S/1
  LAS_SLASwitchStatus_S/1 -> LAS_SLASwitchStatus_1sat/1
  LAS_SLASwitchStatus_1sat/1 -> LAS_SLASwitchStatus_Convert1/1
  LAS_SLASwitchStatus_Convert1/1 -> LAS_SLASwitchStatus_L/1
  LAS_SLASwitchStatus_L/1 -> LAS_SLASwitchStatus_Convert/1
  LAS_SLASwitchStatus_Convert/1 -> output1/1
  Constant2/1 -> output2/1
  Constant3/1 -> output3/1
  Constant4/1 -> output4/1
  Constant5/1 -> output5/1
  Constant6/1 -> output6/1
  Constant7/1 -> output7/1
  Constant8/1 -> output8/1

== system VCU_CS75_12_30_test/长安CS75底盘程序，20ms一次/Output/Subsystem/TransmitMessages10/LAS_29D/LAS_VoiceWarning ==
  LAS_VoiceWarning : Inport
  Constant{1..2,4..8} (7 alike) : Constant  Value=0  OutDataTypeStr=uint8
  LAS_VoiceWarningRon : Rounding  Operator=round
  LAS_VoiceWarning_1sat : Saturate  UpperLimit=192  LowerLimit=0
  LAS_VoiceWarning_Convert : DataTypeConversion  OutDataTypeStr=uint8
  LAS_VoiceWarning_Convert1 : DataTypeConversion  OutDataTypeStr=uint32
  LAS_VoiceWarning_D : Product  Inputs=*/
  LAS_VoiceWarning_F : Constant  OutDataTypeStr=single
  LAS_VoiceWarning_L : simulink/Logic and Bit Operations/Bitwise Operator  logicop=AND  UseBitMask=on  BitMask=192  BitMaskRealWorld=Stored Integer
  LAS_VoiceWarning_O : Constant  Value=0  OutDataTypeStr=single
  LAS_VoiceWarning_S : ArithShift  BitShiftNumber=-6
  LAS_VoiceWarning_sat : Saturate  UpperLimit=0  LowerLimit=0
  LAS_VoiceWarning_st : Sum  Inputs=+-
  output1 : Outport
  output2 : Outport  Port=2
  output3 : Outport  Port=3
  output4 : Outport  Port=4
  output5 : Outport  Port=5
  output6 : Outport  Port=6
  output7 : Outport  Port=7
  output8 : Outport  Port=8
  wires:
  LAS_VoiceWarning/1 -> LAS_VoiceWarning_sat/1
  LAS_VoiceWarning_sat/1 -> LAS_VoiceWarning_st/1
  LAS_VoiceWarning_O/1 -> LAS_VoiceWarning_st/2
  LAS_VoiceWarning_st/1 -> LAS_VoiceWarning_D/1
  LAS_VoiceWarning_F/1 -> LAS_VoiceWarning_D/2
  LAS_VoiceWarning_D/1 -> LAS_VoiceWarningRon/1
  LAS_VoiceWarningRon/1 -> LAS_VoiceWarning_S/1
  LAS_VoiceWarning_S/1 -> LAS_VoiceWarning_1sat/1
  LAS_VoiceWarning_1sat/1 -> LAS_VoiceWarning_Convert1/1
  LAS_VoiceWarning_Convert1/1 -> LAS_VoiceWarning_L/1
  LAS_VoiceWarning_L/1 -> LAS_VoiceWarning_Convert/1
  LAS_VoiceWarning_Convert/1 -> output3/1
  Constant1/1 -> output1/1
  Constant2/1 -> output2/1
  Constant4/1 -> output4/1
  Constant5/1 -> output5/1
  Constant6/1 -> output6/1
  Constant7/1 -> output7/1
  Constant8/1 -> output8/1

== system VCU_CS75_12_30_test/长安CS75底盘程序，20ms一次/Output/Subsystem/TransmitMessages10/LAS_29D/RollingConter ==
  RollingConter : Inport
  Constant{1..6,8} (7 alike) : Constant  Value=0  OutDataTypeStr=uint8
  RollingConterRon : Rounding  Operator=round
  RollingConter_1sat : Saturate  UpperLimit=15  LowerLimit=0
  RollingConter_Convert : DataTypeConversion  OutDataTypeStr=uint8
  RollingConter_Convert1 : DataTypeConversion  OutDataTypeStr=uint32
  RollingConter_D : Product  Inputs=*/
  RollingConter_F : Constant  OutDataTypeStr=single
  RollingConter_L : simulink/Logic and Bit Operations/Bitwise Operator  logicop=AND  UseBitMask=on  BitMask=15  BitMaskRealWorld=Stored Integer
  RollingConter_O : Constant  Value=0  OutDataTypeStr=single
  RollingConter_S : ArithShift
  RollingConter_sat : Saturate  UpperLimit=0  LowerLimit=0
  RollingConter_st : Sum  Inputs=+-
  output1 : Outport
  output2 : Outport  Port=2
  output3 : Outport  Port=3
  output4 : Outport  Port=4
  output5 : Outport  Port=5
  output6 : Outport  Port=6
  output7 : Outport  Port=7
  output8 : Outport  Port=8
  wires:
  RollingConter/1 -> RollingConter_sat/1
  RollingConter_sat/1 -> RollingConter_st/1
  RollingConter_O/1 -> RollingConter_st/2
  RollingConter_st/1 -> RollingConter_D/1
  RollingConter_F/1 -> RollingConter_D/2
  RollingConter_D/1 -> RollingConterRon/1
  RollingConterRon/1 -> RollingConter_S/1
  RollingConter_S/1 -> RollingConter_1sat/1
  RollingConter_1sat/1 -> RollingConter_Convert1/1
  RollingConter_Convert1/1 -> RollingConter_L/1
  RollingConter_L/1 -> RollingConter_Convert/1
  RollingConter_Convert/1 -> output7/1
  Constant1/1 -> output1/1
  Constant2/1 -> output2/1
  Constant3/1 -> output3/1
  Constant4/1 -> output4/1
  Constant5/1 -> output5/1
  Constant6/1 -> output6/1
  Constant8/1 -> output8/1

== system VCU_CS75_12_30_test/长安CS75底盘程序，20ms一次/Output/Subsystem/TransmitMessages11/GW_LCDAL_2EA/LCDAL_AudioWarningEnableStatus ==
  LCDAL_AudioWarningEnableStatus : Inport
  Constant{1..4,6..8} (7 alike) : Constant  Value=0  OutDataTypeStr=uint8
  LCDAL_AudioWarningEnableStatusABS : Abs
  LCDAL_AudioWarningEnableStatusCS : ArithShift  BitShiftNumber=-2
  LCDAL_AudioWarningEnableStatusConS : Constant  OutDataTypeStr=single
  LCDAL_AudioWarningEnableStatusCosR : Constant  Value=0  OutDataTypeStr=uint8
  LCDAL_AudioWarningEnableStatusROP : RelationalOperator  Operator=<  OutDataTypeStr=boolean
  LCDAL_AudioWarningEnableStatusRon : Rounding  Operator=round
  LCDAL_AudioWarningEnableStatusSW : Switch  Criteria=u2 ~= 0
  LCDAL_AudioWarningEnableStatus_1sat : Saturate  UpperLimit=192  LowerLimit=0
  LCDAL_AudioWarningEnableStatus_Convert : DataTypeConversion  OutDataTypeStr=uint8
  LCDAL_AudioWarningEnableStatus_Convert1 : DataTypeConversion  OutDataTypeStr=uint32
  LCDAL_AudioWarningEnableStatus_D : Product  Inputs=*/
  LCDAL_AudioWarningEnableStatus_F : Constant  OutDataTypeStr=single
  LCDAL_AudioWarningEnableStatus_L : simulink/Logic and Bit Operations/Bitwise Operator  logicop=AND  UseBitMask=on  BitMask=192  BitMaskRealWorld=Stored Integer
  LCDAL_AudioWarningEnableStatus_O : Constant  Value=0  OutDataTypeStr=single
  LCDAL_AudioWarningEnableStatus_S : ArithShift  BitShiftNumber=-6
  LCDAL_AudioWarningEnableStatus_sat : Saturate  UpperLimit=3  LowerLimit=0
  LCDAL_AudioWarningEnableStatus_st : Sum  Inputs=+-
  LCDAL_AudioWarningEnableStatussubcon : Sum  Inputs=+-
  output1 : Outport
  output2 : Outport  Port=2
  output3 : Outport  Port=3
  output4 : Outport  Port=4
  output5 : Outport  Port=5
  output6 : Outport  Port=6
  output7 : Outport  Port=7
  output8 : Outport  Port=8
  wires:
  Constant8/1 -> output8/1
  Constant7/1 -> output7/1
  Constant6/1 -> output6/1
  Constant4/1 -> output4/1
  Constant3/1 -> output3/1
  Constant2/1 -> output2/1
  Constant1/1 -> output1/1
  LCDAL_AudioWarningEnableStatus_Convert/1 -> output5/1
  LCDAL_AudioWarningEnableStatus_L/1 -> LCDAL_AudioWarningEnableStatus_Convert/1
  LCDAL_AudioWarningEnableStatus_Convert1/1 -> LCDAL_AudioWarningEnableStatus_L/1
  LCDAL_AudioWarningEnableStatus_1sat/1 -> LCDAL_AudioWarningEnableStatus_Convert1/1
  LCDAL_AudioWarningEnableStatus_S/1 -> LCDAL_AudioWarningEnableStatus_1sat/1
  LCDAL_AudioWarningEnableStatusSW/1 -> LCDAL_AudioWarningEnableStatus_S/1
  LCDAL_AudioWarningEnableStatusROP/1 -> LCDAL_AudioWarningEnableStatusSW/2
  LCDAL_AudioWarningEnableStatussubcon/1 -> LCDAL_AudioWarningEnableStatusSW/1
  LCDAL_AudioWarningEnableStatusABS/1 -> LCDAL_AudioWarningEnableStatussubcon/2
  LCDAL_AudioWarningEnableStatusCS/1 -> LCDAL_AudioWarningEnableStatussubcon/1
  LCDAL_AudioWarningEnableStatusConS/1 -> LCDAL_AudioWarningEnableStatusCS/1
  LCDAL_AudioWarningEnableStatusCosR/1 -> LCDAL_AudioWarningEnableStatusROP/2
  LCDAL_AudioWarningEnableStatusRon/1 -> LCDAL_AudioWarningEnableStatusSW/3, LCDAL_AudioWarningEnableStatusABS/1, LCDAL_AudioWarningEnableStatusROP/1
  LCDAL_AudioWarningEnableStatus_D/1 -> LCDAL_AudioWarningEnableStatusRon/1
  LCDAL_AudioWarningEnableStatus_F/1 -> LCDAL_AudioWarningEnableStatus_D/2
  LCDAL_AudioWarningEnableStatus_st/1 -> LCDAL_AudioWarningEnableStatus_D/1
  LCDAL_AudioWarningEnableStatus_O/1 -> LCDAL_AudioWarningEnableStatus_st/2
  LCDAL_AudioWarningEnableStatus_sat/1 -> LCDAL_AudioWarningEnableStatus_st/1
  LCDAL_AudioWarningEnableStatus/1 -> LCDAL_AudioWarningEnableStatus_sat/1

== system VCU_CS75_12_30_test/长安CS75底盘程序，20ms一次/Output/Subsystem/TransmitMessages11/GW_LCDAL_2EA/LCDAL_BSDLCAAlert ==
  LCDAL_BSDLCAAlert : Inport
  Constant{2..8} (7 alike) : Constant  Value=0  OutDataTypeStr=uint8
  LCDAL_BSDLCAAlertRon : Rounding  Operator=round
  LCDAL_BSDLCAAlert_1sat : Saturate  UpperLimit=48  LowerLimit=0
  LCDAL_BSDLCAAlert_Convert : DataTypeConversion  OutDataTypeStr=uint8
  LCDAL_BSDLCAAlert_Convert1 : DataTypeConversion  OutDataTypeStr=uint32
  LCDAL_BSDLCAAlert_D : Product  Inputs=*/
  LCDAL_BSDLCAAlert_F : Constant  OutDataTypeStr=single
  LCDAL_BSDLCAAlert_L : simulink/Logic and Bit Operations/Bitwise Operator  logicop=AND  UseBitMask=on  BitMask=48  BitMaskRealWorld=Stored Integer
  LCDAL_BSDLCAAlert_O : Constant  Value=0  OutDataTypeStr=single
  LCDAL_BSDLCAAlert_S : ArithShift  BitShiftNumber=-4
  LCDAL_BSDLCAAlert_sat : Saturate  UpperLimit=3  LowerLimit=0
  LCDAL_BSDLCAAlert_st : Sum  Inputs=+-
  output1 : Outport
  output2 : Outport  Port=2
  output3 : Outport  Port=3
  output4 : Outport  Port=4
  output5 : Outport  Port=5
  output6 : Outport  Port=6
  output7 : Outport  Port=7
  output8 : Outport  Port=8
  wires:
  Constant8/1 -> output8/1
  Constant7/1 -> output7/1
  Constant6/1 -> output6/1
  Constant5/1 -> output5/1
  Constant4/1 -> output4/1
  Constant3/1 -> output3/1
  Constant2/1 -> output2/1
  LCDAL_BSDLCAAlert_Convert/1 -> output1/1
  LCDAL_BSDLCAAlert_L/1 -> LCDAL_BSDLCAAlert_Convert/1
  LCDAL_BSDLCAAlert_Convert1/1 -> LCDAL_BSDLCAAlert_L/1
  LCDAL_BSDLCAAlert_1sat/1 -> LCDAL_BSDLCAAlert_Convert1/1
  LCDAL_BSDLCAAlert_S/1 -> LCDAL_BSDLCAAlert_1sat/1
  LCDAL_BSDLCAAlertRon/1 -> LCDAL_BSDLCAAlert_S/1
  LCDAL_BSDLCAAlert_D/1 -> LCDAL_BSDLCAAlertRon/1
  LCDAL_BSDLCAAlert_F/1 -> LCDAL_BSDLCAAlert_D/2
  LCDAL_BSDLCAAlert_st/1 -> LCDAL_BSDLCAAlert_D/1
  LCDAL_BSDLCAAlert_O/1 -> LCDAL_BSDLCAAlert_st/2
  LCDAL_BSDLCAAlert_sat/1 -> LCDAL_BSDLCAAlert_st/1
  LCDAL_BSDLCAAlert/1 -> LCDAL_BSDLCAAlert_sat/1

== system VCU_CS75_12_30_test/长安CS75底盘程序，20ms一次/Output/Subsystem/TransmitMessages11/GW_LCDAL_2EA/LCDAL_BSDLCAEnableStatus ==
  LCDAL_BSDLCAEnableStatus : Inport
  Constant{2..8} (7 alike) : Constant  Value=0  OutDataTypeStr=uint8
  LCDAL_BSDLCAEnableStatusRon : Rounding  Operator=round
  LCDAL_BSDLCAEnableStatus_1sat : Saturate  UpperLimit=192  LowerLimit=0
  LCDAL_BSDLCAEnableStatus_Convert : DataTypeConversion  OutDataTypeStr=uint8
  LCDAL_BSDLCAEnableStatus_Convert1 : DataTypeConversion  OutDataTypeStr=uint32
  LCDAL_BSDLCAEnableStatus_D : Product  Inputs=*/
  LCDAL_BSDLCAEnableStatus_F : Constant  OutDataTypeStr=single
  LCDAL_BSDLCAEnableStatus_L : simulink/Logic and Bit Operations/Bitwise Operator  logicop=AND  UseBitMask=on  BitMask=192  BitMaskRealWorld=Stored Integer
  LCDAL_BSDLCAEnableStatus_O : Constant  Value=0  OutDataTypeStr=single
  LCDAL_BSDLCAEnableStatus_S : ArithShift  BitShiftNumber=-6
  LCDAL_BSDLCAEnableStatus_sat : Saturate  UpperLimit=3  LowerLimit=0
  LCDAL_BSDLCAEnableStatus_st : Sum  Inputs=+-
  output1 : Outport
  output2 : Outport  Port=2
  output3 : Outport  Port=3
  output4 : Outport  Port=4
  output5 : Outport  Port=5
  output6 : Outport  Port=6
  output7 : Outport  Port=7
  output8 : Outport  Port=8
  wires:
  Constant8/1 -> output8/1
  Constant7/1 -> output7/1
  Constant6/1 -> output6/1
  Constant5/1 -> output5/1
  Constant4/1 -> output4/1
  Constant3/1 -> output3/1
  Constant2/1 -> output2/1
  LCDAL_BSDLCAEnableStatus_Convert/1 -> output1/1
  LCDAL_BSDLCAEnableStatus_L/1 -> LCDAL_BSDLCAEnableStatus_Convert/1
  LCDAL_BSDLCAEnableStatus_Convert1/1 -> LCDAL_BSDLCAEnableStatus_L/1
  LCDAL_BSDLCAEnableStatus_1sat/1 -> LCDAL_BSDLCAEnableStatus_Convert1/1
  LCDAL_BSDLCAEnableStatus_S/1 -> LCDAL_BSDLCAEnableStatus_1sat/1
  LCDAL_BSDLCAEnableStatusRon/1 -> LCDAL_BSDLCAEnableStatus_S/1
  LCDAL_BSDLCAEnableStatus_D/1 -> LCDAL_BSDLCAEnableStatusRon/1
  LCDAL_BSDLCAEnableStatus_F/1 -> LCDAL_BSDLCAEnableStatus_D/2
  LCDAL_BSDLCAEnableStatus_st/1 -> LCDAL_BSDLCAEnableStatus_D/1
  LCDAL_BSDLCAEnableStatus_O/1 -> LCDAL_BSDLCAEnableStatus_st/2
  LCDAL_BSDLCAEnableStatus_sat/1 -> LCDAL_BSDLCAEnableStatus_st/1
  LCDAL_BSDLCAEnableStatus/1 -> LCDAL_BSDLCAEnableStatus_sat/1

== system VCU_CS75_12_30_test/长安CS75底盘程序，20ms一次/Output/Subsystem/TransmitMessages11/GW_LCDAL_2EA/LCDAL_BSDLCAStatus ==
  LCDAL_BSDLCAStatus : Inport
  Constant{1,3..8} (7 alike) : Constant  Value=0  OutDataTypeStr=uint8
  LCDAL_BSDLCAStatusRon : Rounding  Operator=round
  LCDAL_BSDLCAStatus_1sat : Saturate  UpperLimit=24  LowerLimit=0
  LCDAL_BSDLCAStatus_Convert : DataTypeConversion  OutDataTypeStr=uint8
  LCDAL_BSDLCAStatus_Convert1 : DataTypeConversion  OutDataTypeStr=uint32
  LCDAL_BSDLCAStatus_D : Product  Inputs=*/
  LCDAL_BSDLCAStatus_F : Constant  OutDataTypeStr=single
  LCDAL_BSDLCAStatus_L : simulink/Logic and Bit Operations/Bitwise Operator  logicop=AND  UseBitMask=on  BitMask=24  BitMaskRealWorld=Stored Integer
  LCDAL_BSDLCAStatus_O : Constant  Value=0  OutDataTypeStr=single
  LCDAL_BSDLCAStatus_S : ArithShift  BitShiftNumber=-3
  LCDAL_BSDLCAStatus_sat : Saturate  UpperLimit=3  LowerLimit=0
  LCDAL_BSDLCAStatus_st : Sum  Inputs=+-
  output1 : Outport
  output2 : Outport  Port=2
  output3 : Outport  Port=3
  output4 : Outport  Port=4
  output5 : Outport  Port=5
  output6 : Outport  Port=6
  output7 : Outport  Port=7
  output8 : Outport  Port=8
  wires:
  Constant8/1 -> output8/1
  Constant7/1 -> output7/1
  Constant6/1 -> output6/1
  Constant5/1 -> output5/1
  Constant4/1 -> output4/1
  Constant3/1 -> output3/1
  Constant1/1 -> output1/1
  LCDAL_BSDLCAStatus_Convert/1 -> output2/1
  LCDAL_BSDLCAStatus_L/1 -> LCDAL_BSDLCAStatus_Convert/1
  LCDAL_BSDLCAStatus_Convert1/1 -> LCDAL_BSDLCAStatus_L/1
  LCDAL_BSDLCAStatus_1sat/1 -> LCDAL_BSDLCAStatus_Convert1/1
  LCDAL_BSDLCAStatus_S/1 -> LCDAL_BSDLCAStatus_1sat/1
  LCDAL_BSDLCAStatusRon/1 -> LCDAL_BSDLCAStatus_S/1
  LCDAL_BSDLCAStatus_D/1 -> LCDAL_BSDLCAStatusRon/1
  LCDAL_BSDLCAStatus_F/1 -> LCDAL_BSDLCAStatus_D/2
  LCDAL_BSDLCAStatus_st/1 -> LCDAL_BSDLCAStatus_D/1
  LCDAL_BSDLCAStatus_O/1 -> LCDAL_BSDLCAStatus_st/2
  LCDAL_BSDLCAStatus_sat/1 -> LCDAL_BSDLCAStatus_st/1
  LCDAL_BSDLCAStatus/1 -> LCDAL_BSDLCAStatus_sat/1
